simulink model "DDCU_wxt_v03"  (R2014a)
settings: Solver=ode45  StartTime=0.0  StopTime=50  FixedStep=0.0005  RelTol=1e-3
values from neighbouring files (symbols this model uses):
  ag_thr = 0.4*g    (= 3.924)    [Veh_Par_wxt.m]
  B = 2.25    [Veh_Par_wxt.m]
  bra_pre_em = 12    [Veh_Par_wxt.m]
  bra_pre_gz2 = 12/3    (= 4)    [Veh_Par_wxt.m]
  bra_pre_gz34 = 12/3    (= 4)    [Veh_Par_wxt.m]
  bra_pre_yd = 12/2    (= 6)    [Veh_Par_wxt.m]
  brakepre_dem_data = [0 1 2 3 4 5 6 7 8 9 10 11 12]    [Veh_Par_wxt.m]
  brakeTrq_dem_data = [0 218.198 436.396 654.594 872.792 1090.99 1309.188 1527.386 1745.584 1963.782 2181.98 2400.178 2618.376]    [Veh_Par_wxt.m]
  bratrq_max = 4*2618.376    (= 10473.504)    [Veh_Par_wxt.m]
  eff_tran = 0.75    [Veh_Par_wxt.m]
  G = Mass*g    (= 36297)    [Veh_Par_wxt.m]
  kd1 = 1    [Veh_Par_wxt.m]
  kd2 = 1    [Veh_Par_wxt.m]
  kd3 = 1    [Veh_Par_wxt.m]
  ki1 = 1    [Veh_Par_wxt.m]
  ki2 = 1    [Veh_Par_wxt.m]
  ki3 = 1    [Veh_Par_wxt.m]
  kp1 = 1    [Veh_Par_wxt.m]
  kp2 = 1    [Veh_Par_wxt.m]
  kp3 = 1    [Veh_Par_wxt.m]
  L = 3.12    [Veh_Par_wxt.m]
  premax = 12    [Veh_Par_wxt.m]
  Radius = 0.20    (= 0.2)    [Veh_Par_wxt.m]
  s_opt_yi_add = 0.05    [Veh_Par_wxt.m]
  s_opt_zhuan_add = 0.05    [Veh_Par_wxt.m]
  spd_map_mot = [0 100 200 300 360 400 500 600 700 800 900]*tras_ratio    [Veh_Par_wxt.m]
  spdmax = 900*tras_ratio    (= 5580)    [Veh_Par_wxt.m]
  speed_thr_park = 5/3.6/Radius*30/pi    (= 66.3145596216)    [Veh_Par_wxt.m]
  tras_ratio = 6.2    [Veh_Par_wxt.m]
  trq_map_mot = [1200 1200 1200 1200 1200 1080 864 720 617 540 480]/tras_ratio    [Veh_Par_wxt.m]
  trqmax = 80    [Veh_Par_wxt.m]
  v_thr1_b = 5    [Veh_Par_wxt.m]
  v_thr2_b = 20    [Veh_Par_wxt.m]
  v_thr_park = 5    [Veh_Par_wxt.m]
undefined symbols (not defined in the file or in its folder): DiscIntNeverNeededParam
libraries: simulink x34, Solver_SF x1
(part 6 of 10)

== system DDCU_wxt_v03/MainControl/mode_control/backward/backward/Drive/驱动防滑控制TCS/转向TCS/右转 ==
  trq_dem_lf : Inport
  trq_dem_lr : Inport  Port=2
  trq_dem_rf : Inport  Port=3
  trq_dem_rr : Inport  Port=4
  bra_pre_l : Inport  Port=5
  bra_pre_r : Inport  Port=6
  s_act_lf : Inport  Port=7
  s_act_lr : Inport  Port=8
  s_act_rf : Inport  Port=9
  s_act_rr : Inport  Port=10
  brake_dem : Inport  Port=11
  s_opt_zhuan : Inport  Port=12
  Action Port : ActionPort
  Constant{,1..3} (4 alike) : Constant  Value=s_opt_zhuan_add
  MATLAB Function : MATLAB Function  TreatAsAtomicUnit=on
  MATLAB Function1 : MATLAB Function  TreatAsAtomicUnit=on
  MATLAB Function2 : MATLAB Function  TreatAsAtomicUnit=on
  MATLAB Function3 : MATLAB Function  TreatAsAtomicUnit=on
  MATLAB Function4 : MATLAB Function  TreatAsAtomicUnit=on
  Memory{,1..3} (4 alike) : Memory  InheritSampleTime=on
  Multiport Switch : MultiPortSwitch  DataPortOrder=Zero-based contiguous  Inputs=4
  Mux{,1..3} (4 alike) : Mux  Inputs=6
  Switch Case : SwitchCase  CaseConditions={0,1,2,3}  ShowDefaultCase=off
  Terminator : Terminator
  Terminator1 : Terminator
  前后轮均滑转 : Subsystem  TreatAsAtomicUnit=on
  前轮滑转 : Subsystem  TreatAsAtomicUnit=on
  后轮滑转 : Subsystem  TreatAsAtomicUnit=on
  无滑转 : Subsystem  TreatAsAtomicUnit=on
  backward_dem : Outport
  wires:
  s_act_lf/1 -> MATLAB Function/1(s_act_lf), [s_act_lf]
  MATLAB Function/1(flag_lf) -> Memory/1, [flag_lf]
  Memory/1 -> MATLAB Function/4(flag_lf_pre)
  Constant/1 -> MATLAB Function/3(s_opt_zhuan_add)
  s_act_lr/1 -> MATLAB Function1/1(s_act_lr), [s_act_lr]
  MATLAB Function1/1(flag_lr) -> [flag_lr], Memory1/1
  Memory1/1 -> MATLAB Function1/4(flag_lr_pre)
  Constant1/1 -> MATLAB Function1/3(s_opt_zhuan_add)
  s_act_rf/1 -> MATLAB Function2/1(s_act_rf)
  MATLAB Function2/1(flag_rf) -> Memory2/1, Terminator/1
  Memory2/1 -> MATLAB Function2/4(flag_rf_pre)
  Constant2/1 -> MATLAB Function2/3(s_opt_zhuan_add)
  s_act_rr/1 -> MATLAB Function3/1(s_act_rr)
  s_opt_zhuan/1 -> [s_opt_zhuan], MATLAB Function3/2(s_opt_zhuan), MATLAB Function2/2(s_opt_zhuan), MATLAB Function1/2(s_opt_zhuan), MATLAB Function/2(s_opt_zhuan)
  MATLAB Function3/1(flag_rr) -> Memory3/1, Terminator1/1
  Memory3/1 -> MATLAB Function3/4(flag_rr_pre)
  Constant3/1 -> MATLAB Function3/3(s_opt_zhuan_add)
  [flag_lf] -> MATLAB Function4/1(flag_lf)
  [flag_lr] -> MATLAB Function4/2(flag_lr)
  MATLAB Function4/1(y) -> Multiport Switch/1, Switch Case/1
  Switch Case/1 -> 无滑转/Action
  trq_dem_lf/1 -> 无滑转/1(trq_dem_lf), 前后轮均滑转/1(trq_dem_lf), 后轮滑转/1(trq_dem_lf), 前轮滑转/1(trq_dem_lf)
  trq_dem_lr/1 -> 无滑转/2(trq_dem_lr), 前轮滑转/2(trq_dem_lr), 前后轮均滑转/2(trq_dem_lr), 后轮滑转/2(trq_dem_lr)
  trq_dem_rf/1 -> 无滑转/3(trq_dem_rf), 前后轮均滑转/3(trq_dem_rf), 后轮滑转/3(trq_dem_rf), 前轮滑转/3(trq_dem_rf)
  trq_dem_rr/1 -> 无滑转/4(trq_dem_rr), 前后轮均滑转/4(trq_dem_rr), 后轮滑转/4(trq_dem_rr), 前轮滑转/4(trq_dem_rr)
  bra_pre_l/1 -> 无滑转/5(bra_pre_l), 前后轮均滑转/5(bra_pre_l), 后轮滑转/5(bra_pre_l), 前轮滑转/5(bra_pre_l)
  bra_pre_r/1 -> 无滑转/6(bra_pre_r), 前后轮均滑转/6(bra_pre_r), 后轮滑转/6(bra_pre_r), 前轮滑转/6(bra_pre_r)
  brake_dem/1 -> 无滑转/7(brake_dem), 前后轮均滑转/7(brake_dem), 后轮滑转/7(brake_dem), 前轮滑转/7(brake_dem)
  无滑转/1(mot_lf) -> Mux/1
  无滑转/2(mot_lr) -> Mux/2
  无滑转/4(mot_rr) -> Mux/4
  无滑转/3(mot_rf) -> Mux/3
  无滑转/5(bra_pre_l1) -> Mux/5
  无滑转/6(bra_pre_r1) -> Mux/6
  Mux/1 -> Multiport Switch/2
  Multiport Switch/1 -> backward_dem/1
  Switch Case/2 -> 前轮滑转/Action
  前轮滑转/6(bra_pre_r1) -> Mux1/6
  前轮滑转/3(mot_rf) -> Mux1/3
  前轮滑转/2(mot_lr) -> Mux1/2
  前轮滑转/1(mot_lf) -> Mux1/1
  前轮滑转/5(bra_pre_l1) -> Mux1/5
  前轮滑转/4(mot_rr) -> Mux1/4
  Mux1/1 -> Multiport Switch/3
  [s_act_lf] -> 前轮滑转/8(s_act_lf)
  [s_opt_zhuan] -> 前轮滑转/9(s_opt_zhuan)
  后轮滑转/1(mot_lf) -> Mux2/1
  后轮滑转/3(mot_rf) -> Mux2/3
  后轮滑转/2(mot_lr) -> Mux2/2
  后轮滑转/4(mot_rr) -> Mux2/4
  后轮滑转/5(bra_pre_l1) -> Mux2/5
  后轮滑转/6(bra_pre_r1) -> Mux2/6
  Mux2/1 -> Multiport Switch/4
  [s_act_lr] -> 后轮滑转/8(s_act_lr)
  [s_opt_zhuan] -> 后轮滑转/9(s_opt_zhuan)
  Switch Case/3 -> 后轮滑转/Action
  前后轮均滑转/1(mot_lf) -> Mux3/1
  前后轮均滑转/3(mot_rf) -> Mux3/3
  前后轮均滑转/2(mot_lr) -> Mux3/2
  前后轮均滑转/4(mot_rr) -> Mux3/4
  前后轮均滑转/5(bra_pre_l1) -> Mux3/5
  前后轮均滑转/6(bra_pre_r1) -> Mux3/6
  Switch Case/4 -> 前后轮均滑转/Action
  [s_act_lf] -> 前后轮均滑转/8(s_act_lf)
  [s_act_lr] -> 前后轮均滑转/9(s_act_lr)
  [s_opt_zhuan] -> 前后轮均滑转/10(s_opt_zhuan)
  Mux3/1 -> Multiport Switch/5

== system DDCU_wxt_v03/MainControl/mode_control/backward/backward/Drive/驱动防滑控制TCS/转向TCS/左转 ==
  trq_dem_lf : Inport
  trq_dem_lr : Inport  Port=2
  trq_dem_rf : Inport  Port=3
  trq_dem_rr : Inport  Port=4
  bra_pre_l : Inport  Port=5
  bra_pre_r : Inport  Port=6
  s_act_lf : Inport  Port=7
  s_act_lr : Inport  Port=8
  s_act_rf : Inport  Port=9
  s_act_rr : Inport  Port=10
  brake_dem : Inport  Port=11
  s_opt_zhuan : Inport  Port=12
  Action Port : ActionPort
  Constant{,1..3} (4 alike) : Constant  Value=s_opt_zhuan_add
  MATLAB Function : MATLAB Function  TreatAsAtomicUnit=on
  MATLAB Function1 : MATLAB Function  TreatAsAtomicUnit=on
  MATLAB Function2 : MATLAB Function  TreatAsAtomicUnit=on
  MATLAB Function3 : MATLAB Function  TreatAsAtomicUnit=on
  MATLAB Function4 : MATLAB Function  TreatAsAtomicUnit=on
  Memory{,1..3} (4 alike) : Memory  InheritSampleTime=on
  Multiport Switch : MultiPortSwitch  DataPortOrder=Zero-based contiguous  Inputs=4
  Mux{,1..3} (4 alike) : Mux  Inputs=6
  Switch Case : SwitchCase  CaseConditions={0,1,2,3}  ShowDefaultCase=off
  Terminator : Terminator
  Terminator1 : Terminator
  前后轮均滑转 : Subsystem  TreatAsAtomicUnit=on
  前轮滑转 : Subsystem  TreatAsAtomicUnit=on
  后轮滑转 : Subsystem  TreatAsAtomicUnit=on
  无滑转 : Subsystem  TreatAsAtomicUnit=on
  backward_dem : Outport
  wires:
  Mux3/1 -> Multiport Switch/5
  [s_opt_zhuan] -> 前后轮均滑转/10(s_opt_zhuan)
  [s_act_rr] -> 前后轮均滑转/9(s_act_rr)
  [s_act_rf] -> 前后轮均滑转/8(s_act_rf)
  Switch Case/4 -> 前后轮均滑转/Action
  前后轮均滑转/6(bra_pre_r1) -> Mux3/6
  前后轮均滑转/5(bra_pre_l1) -> Mux3/5
  前后轮均滑转/4(mot_rr) -> Mux3/4
  前后轮均滑转/2(mot_lr) -> Mux3/2
  前后轮均滑转/3(mot_rf) -> Mux3/3
  前后轮均滑转/1(mot_lf) -> Mux3/1
  Switch Case/3 -> 后轮滑转/Action
  [s_opt_zhuan] -> 后轮滑转/9(s_opt_zhuan)
  [s_act_rr] -> 后轮滑转/8(s_act_rr)
  Mux2/1 -> Multiport Switch/4
  后轮滑转/6(bra_pre_r1) -> Mux2/6
  后轮滑转/5(bra_pre_l1) -> Mux2/5
  后轮滑转/4(mot_rr) -> Mux2/4
  后轮滑转/2(mot_lr) -> Mux2/2
  后轮滑转/3(mot_rf) -> Mux2/3
  后轮滑转/1(mot_lf) -> Mux2/1
  [s_opt_zhuan] -> 前轮滑转/9(s_opt_zhuan)
  [s_act_rf] -> 前轮滑转/8(s_act_rf)
  Mux1/1 -> Multiport Switch/3
  前轮滑转/4(mot_rr) -> Mux1/4
  前轮滑转/5(bra_pre_l1) -> Mux1/5
  前轮滑转/1(mot_lf) -> Mux1/1
  前轮滑转/2(mot_lr) -> Mux1/2
  前轮滑转/3(mot_rf) -> Mux1/3
  前轮滑转/6(bra_pre_r1) -> Mux1/6
  Switch Case/2 -> 前轮滑转/Action
  Multiport Switch/1 -> backward_dem/1
  Mux/1 -> Multiport Switch/2
  无滑转/6(bra_pre_r1) -> Mux/6
  无滑转/5(bra_pre_l1) -> Mux/5
  无滑转/3(mot_rf) -> Mux/3
  无滑转/4(mot_rr) -> Mux/4
  无滑转/2(mot_lr) -> Mux/2
  无滑转/1(mot_lf) -> Mux/1
  brake_dem/1 -> 前轮滑转/7(brake_dem), 后轮滑转/7(brake_dem), 前后轮均滑转/7(brake_dem), 无滑转/7(brake_dem)
  bra_pre_r/1 -> 前轮滑转/6(bra_pre_r), 后轮滑转/6(bra_pre_r), 前后轮均滑转/6(bra_pre_r), 无滑转/6(bra_pre_r)
  bra_pre_l/1 -> 前轮滑转/5(bra_pre_l), 后轮滑转/5(bra_pre_l), 前后轮均滑转/5(bra_pre_l), 无滑转/5(bra_pre_l)
  trq_dem_rr/1 -> 前轮滑转/4(trq_dem_rr), 后轮滑转/4(trq_dem_rr), 前后轮均滑转/4(trq_dem_rr), 无滑转/4(trq_dem_rr)
  trq_dem_rf/1 -> 前轮滑转/3(trq_dem_rf), 后轮滑转/3(trq_dem_rf), 前后轮均滑转/3(trq_dem_rf), 无滑转/3(trq_dem_rf)
  trq_dem_lr/1 -> 后轮滑转/2(trq_dem_lr), 前后轮均滑转/2(trq_dem_lr), 前轮滑转/2(trq_dem_lr), 无滑转/2(trq_dem_lr)
  trq_dem_lf/1 -> 前轮滑转/1(trq_dem_lf), 后轮滑转/1(trq_dem_lf), 前后轮均滑转/1(trq_dem_lf), 无滑转/1(trq_dem_lf)
  Switch Case/1 -> 无滑转/Action
  MATLAB Function4/1(y) -> Switch Case/1, Multiport Switch/1
  [flag_rr] -> MATLAB Function4/2(flag_rr)
  [flag_rf] -> MATLAB Function4/1(flag_rf)
  Constant3/1 -> MATLAB Function3/3(s_opt_zhuan_add)
  Memory3/1 -> MATLAB Function3/4(flag_rr_pre)
  MATLAB Function3/1(flag_rr) -> Memory3/1, [flag_rr]
  s_opt_zhuan/1 -> MATLAB Function/2(s_opt_zhuan), MATLAB Function1/2(s_opt_zhuan), MATLAB Function2/2(s_opt_zhuan), MATLAB Function3/2(s_opt_zhuan), [s_opt_zhuan]
  s_act_rr/1 -> MATLAB Function3/1(s_act_rr), [s_act_rr]
  Constant2/1 -> MATLAB Function2/3(s_opt_zhuan_add)
  Memory2/1 -> MATLAB Function2/4(flag_rf_pre)
  MATLAB Function2/1(flag_rf) -> [flag_rf], Memory2/1
  s_act_rf/1 -> MATLAB Function2/1(s_act_rf), [s_act_rf]
  Constant1/1 -> MATLAB Function1/3(s_opt_zhuan_add)
  Memory1/1 -> MATLAB Function1/4(flag_lr_pre)
  MATLAB Function1/1(flag_lr) -> Memory1/1, Terminator1/1
  s_act_lr/1 -> MATLAB Function1/1(s_act_lr)
  Constant/1 -> MATLAB Function/3(s_opt_zhuan_add)
  Memory/1 -> MATLAB Function/4(flag_lf_pre)
  MATLAB Function/1(flag_lf) -> Memory/1, Terminator/1
  s_act_lf/1 -> MATLAB Function/1(s_act_lf)

== system DDCU_wxt_v03/MainControl/mode_control/forward/forward/Drive/驱动防滑控制TCS/直行TCS/Subsystem ==
  speed_act_lf : Inport
  v_act : Inport  Port=2
  Add : Sum
  Constant : Constant  Value=eps
  Divide : Product  Inputs=*/
  Gain : Gain  Gain=pi/30
  Gain1 : Gain  Gain=Radius
  Gain2 : Gain  Gain=1/3.6
  Subtract : Sum  Inputs=+-
  s_act_lf : Outport
  wires:
  Divide/1 -> s_act_lf/1
  Add/1 -> Divide/2
  Constant/1 -> Add/2
  Subtract/1 -> Divide/1
  Gain2/1 -> Subtract/2
  Gain1/1 -> Subtract/1, Add/1
  v_act/1 -> Gain2/1
  Gain/1 -> Gain1/1
  speed_act_lf/1 -> Gain/1

== system DDCU_wxt_v03/MainControl/mode_control/forward/forward/Drive/驱动防滑控制TCS/直行TCS/Subsystem1 ==
  speed_act_lr : Inport
  v_act : Inport  Port=2
  Add : Sum
  Constant : Constant  Value=eps
  Divide : Product  Inputs=*/
  Gain : Gain  Gain=pi/30
  Gain1 : Gain  Gain=Radius
  Gain2 : Gain  Gain=1/3.6
  Subtract : Sum  Inputs=+-
  s_act_lr : Outport
  wires:
  speed_act_lr/1 -> Gain/1
  Gain/1 -> Gain1/1
  v_act/1 -> Gain2/1
  Gain1/1 -> Add/1, Subtract/1
  Gain2/1 -> Subtract/2
  Subtract/1 -> Divide/1
  Constant/1 -> Add/2
  Add/1 -> Divide/2
  Divide/1 -> s_act_lr/1

== system DDCU_wxt_v03/MainControl/mode_control/forward/forward/Drive/驱动防滑控制TCS/直行TCS/Subsystem2 ==
  speed_act_rf : Inport
  v_act : Inport  Port=2
  Add : Sum
  Constant : Constant  Value=eps
  Divide : Product  Inputs=*/
  Gain : Gain  Gain=pi/30
  Gain1 : Gain  Gain=Radius
  Gain2 : Gain  Gain=1/3.6
  Subtract : Sum  Inputs=+-
  s_act_rf : Outport
  wires:
  Divide/1 -> s_act_rf/1
  Add/1 -> Divide/2
  Constant/1 -> Add/2
  Subtract/1 -> Divide/1
  Gain2/1 -> Subtract/2
  Gain1/1 -> Subtract/1, Add/1
  v_act/1 -> Gain2/1
  Gain/1 -> Gain1/1
  speed_act_rf/1 -> Gain/1

== system DDCU_wxt_v03/MainControl/mode_control/forward/forward/Drive/驱动防滑控制TCS/直行TCS/Subsystem3 ==
  speed_act_rr : Inport
  v_act : Inport  Port=2
  Add : Sum
  Constant : Constant  Value=eps
  Divide : Product  Inputs=*/
  Gain : Gain  Gain=pi/30
  Gain1 : Gain  Gain=Radius
  Gain2 : Gain  Gain=1/3.6
  Subtract : Sum  Inputs=+-
  s_act_rr : Outport
  wires:
  speed_act_rr/1 -> Gain/1
  Gain/1 -> Gain1/1
  v_act/1 -> Gain2/1
  Gain1/1 -> Add/1, Subtract/1
  Gain2/1 -> Subtract/2
  Subtract/1 -> Divide/1
  Constant/1 -> Add/2
  Add/1 -> Divide/2
  Divide/1 -> s_act_rr/1

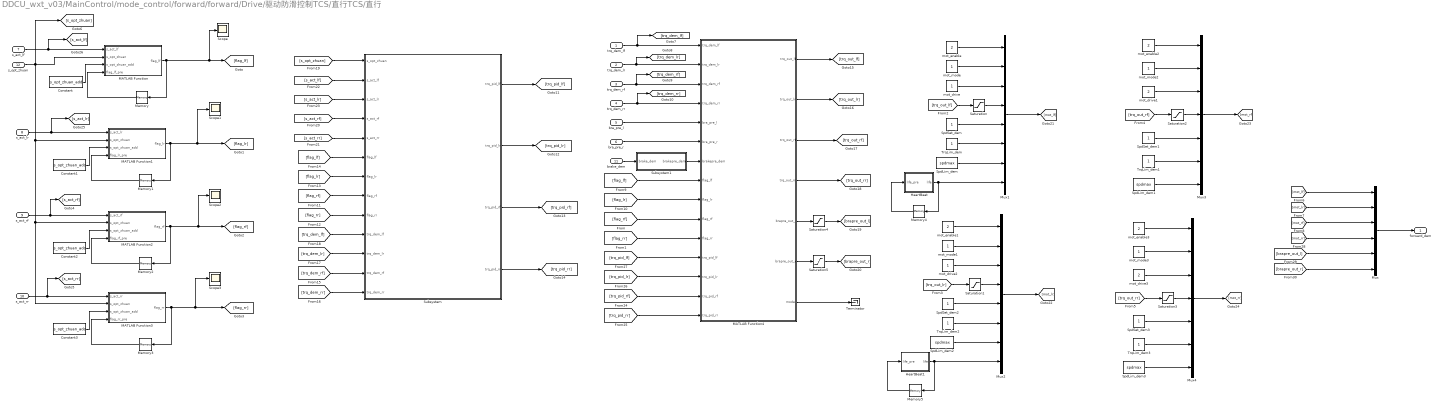
== system DDCU_wxt_v03/MainControl/mode_control/forward/forward/Drive/驱动防滑控制TCS/直行TCS/直行 ==
  trq_dem_lf : Inport
  trq_dem_lr : Inport  Port=2
  trq_dem_rf : Inport  Port=3
  trq_dem_rr : Inport  Port=4
  bra_pre_l : Inport  Port=5
  bra_pre_r : Inport  Port=6
  s_act_lf : Inport  Port=7
  s_act_lr : Inport  Port=8
  s_act_rf : Inport  Port=9
  s_act_rr : Inport  Port=10
  brake_dem : Inport  Port=11
  s_opt_zhuan : Inport  Port=12
  Constant{,1..3} (4 alike) : Constant  Value=s_opt_zhuan_add
  HeartBeat : MATLAB Function  TreatAsAtomicUnit=on
  HeartBeat1 : MATLAB Function  TreatAsAtomicUnit=on
  MATLAB Function : MATLAB Function  TreatAsAtomicUnit=on
  MATLAB Function1 : MATLAB Function  TreatAsAtomicUnit=on
  MATLAB Function2 : MATLAB Function  TreatAsAtomicUnit=on
  MATLAB Function3 : MATLAB Function  TreatAsAtomicUnit=on
  MATLAB Function4 : MATLAB Function  TreatAsAtomicUnit=on
  Memory{,1..5} (6 alike) : Memory  InheritSampleTime=on
  Mux : Mux  Inputs=6
  Mux1 : Mux  Inputs=8
  Mux2 : Mux  Inputs=8
  Mux3 : Mux  Inputs=7
  Mux4 : Mux  Inputs=7
  Saturation{,1..3} (4 alike) : Saturate  UpperLimit=trqmax  LowerLimit=0
  Saturation4 : Saturate  UpperLimit=premax  LowerLimit=0
  Saturation5 : Saturate  UpperLimit=premax  LowerLimit=0
  Scope{,1..3} (4 alike) : Scope
      Scope settings: SaveName=ScopeData43
      Scope1 settings: SaveName=ScopeData44
      Scope2 settings: SaveName=ScopeData45
      Scope3 settings: SaveName=ScopeData46
  SpdLim_dem{,1..3} (4 alike) : Constant  Value=spdmax
  SpdSet_dem{,1..3} (4 alike) : Constant
  Subsystem : Subsystem
  Subsystem1 : Subsystem
  Terminator : Terminator
  TrqLim_dem{,1..3} (4 alike) : Constant
  mot_drive : Constant
  mot_drive1 : Constant  Value=2
  mot_drive2 : Constant
  mot_drive3 : Constant  Value=2
  mot_enable{,1..3} (4 alike) : Constant  Value=2
  mot_mode{,1..3} (4 alike) : Constant
  forward_dem : Outport
  wires:
  Mux/1 -> forward_dem/1
  [flag_rr] -> MATLAB Function4/11(flag_rr)
  [flag_rf] -> MATLAB Function4/10(flag_rf)
  Constant3/1 -> MATLAB Function3/3(s_opt_zhuan_add)
  Memory3/1 -> MATLAB Function3/4(flag_rr_pre)
  MATLAB Function3/1(flag_rr) -> Memory3/1, Scope3/1, [flag_rr]
  s_opt_zhuan/1 -> MATLAB Function/2(s_opt_zhuan), MATLAB Function1/2(s_opt_zhuan), MATLAB Function2/2(s_opt_zhuan), MATLAB Function3/2(s_opt_zhuan), [s_opt_zhuan]
  s_act_rr/1 -> MATLAB Function3/1(s_act_rr), [s_act_rr]
  Constant2/1 -> MATLAB Function2/3(s_opt_zhuan_add)
  Memory2/1 -> MATLAB Function2/4(flag_rf_pre)
  MATLAB Function2/1(flag_rf) -> Scope2/1, [flag_rf], Memory2/1
  s_act_rf/1 -> MATLAB Function2/1(s_act_rf), [s_act_rf]
  Constant1/1 -> MATLAB Function1/3(s_opt_zhuan_add)
  Memory1/1 -> MATLAB Function1/4(flag_lr_pre)
  MATLAB Function1/1(flag_lr) -> Memory1/1, Scope1/1, [flag_lr]
  s_act_lr/1 -> [s_act_lr], MATLAB Function1/1(s_act_lr)
  Constant/1 -> MATLAB Function/3(s_opt_zhuan_add)
  Memory/1 -> MATLAB Function/4(flag_lf_pre)
  MATLAB Function/1(flag_lf) -> Scope/1, [flag_lf], Memory/1
  s_act_lf/1 -> [s_act_lf], MATLAB Function/1(s_act_lf)
  [flag_lr] -> MATLAB Function4/9(flag_lr)
  [flag_lf] -> MATLAB Function4/8(flag_lf)
  [trq_dem_lf] -> Subsystem/10(trq_dem_lf)
  [flag_lf] -> Subsystem/6(flag_lf)
  [trq_dem_rf] -> Subsystem/12(trq_dem_rf)
  [trq_dem_lr] -> Subsystem/11(trq_dem_lr)
  [flag_lr] -> Subsystem/7(flag_lr)
  [flag_rf] -> Subsystem/8(flag_rf)
  [trq_dem_rr] -> Subsystem/13(trq_dem_rr)
  [flag_rr] -> Subsystem/9(flag_rr)
  [s_opt_zhuan] -> Subsystem/1(s_opt_zhuan)
  [s_act_rr] -> Subsystem/5(s_act_rr)
  [s_act_rf] -> Subsystem/4(s_act_rf)
  [s_act_lr] -> Subsystem/3(s_act_lr)
  [s_act_lf] -> Subsystem/2(s_act_lf)
  Subsystem/2(trq_pid_lr) -> [trq_pid_lr]
  Subsystem/1(trq_pid_lf) -> [trq_pid_lf]
  Subsystem/4(trq_pid_rr) -> [trq_pid_rr]
  Subsystem/3(trq_pid_rf) -> [trq_pid_rf]
  [trq_pid_lf] -> MATLAB Function4/12(trq_pid_lf)
  [trq_pid_lr] -> MATLAB Function4/13(trq_pid_lr)
  [trq_pid_rf] -> MATLAB Function4/14(trq_pid_rf)
  [trq_pid_rr] -> MATLAB Function4/15(trq_pid_rr)
  trq_dem_lf/1 -> MATLAB Function4/1(trq_dem_lf), [trq_dem_lf]
  trq_dem_lr/1 -> MATLAB Function4/2(trq_dem_lr), [trq_dem_lr]
  trq_dem_rf/1 -> MATLAB Function4/3(trq_dem_rf), [trq_dem_rf]
  trq_dem_rr/1 -> MATLAB Function4/4(trq_dem_rr), [trq_dem_rr]
  bra_pre_l/1 -> MATLAB Function4/5(bra_pre_l)
  bra_pre_r/1 -> MATLAB Function4/6(bra_pre_r)
  SpdLim_dem3/1 -> Mux4/7
  TrqLim_dem3/1 -> Mux4/6
  Mux4/1 -> [mot_rr]
  SpdSet_dem3/1 -> Mux4/5
  mot_enable3/1 -> Mux4/1
  [trq_out_rr] -> Saturation3/1
  mot_mode3/1 -> Mux4/2
  mot_drive3/1 -> Mux4/3
  SpdLim_dem2/1 -> Mux2/7
  Memory5/1 -> HeartBeat1/1(life_pre)
  HeartBeat1/1(life) -> Memory5/1, Mux2/8
  TrqLim_dem2/1 -> Mux2/6
  Mux2/1 -> [mot_lr]
  SpdSet_dem2/1 -> Mux2/5
  mot_enable1/1 -> Mux2/1
  [trq_out_lr] -> Saturation1/1
  mot_mode1/1 -> Mux2/2
  mot_drive2/1 -> Mux2/3
  SpdLim_dem1/1 -> Mux3/7
  TrqLim_dem1/1 -> Mux3/6
  Mux3/1 -> [mot_rf]
  SpdSet_dem1/1 -> Mux3/5
  mot_enable2/1 -> Mux3/1
  [trq_out_rf] -> Saturation2/1
  mot_mode2/1 -> Mux3/2
  mot_drive1/1 -> Mux3/3
  SpdLim_dem/1 -> Mux1/7
  Memory4/1 -> HeartBeat/1(life_pre)
  HeartBeat/1(life) -> Memory4/1, Mux1/8
  TrqLim_dem/1 -> Mux1/6
  Mux1/1 -> [mot_lf]
  SpdSet_dem/1 -> Mux1/5
  mot_enable/1 -> Mux1/1
  [trq_out_lf] -> Saturation/1
  mot_mode/1 -> Mux1/2
  mot_drive/1 -> Mux1/3
  MATLAB Function4/1(trq_out_lf) -> [trq_out_lf]
  MATLAB Function4/2(trq_out_lr) -> [trq_out_lr]
  MATLAB Function4/3(trq_out_rf) -> [trq_out_rf]
  MATLAB Function4/4(trq_out_rr) -> [trq_out_rr]
  MATLAB Function4/5(brapre_out_l) -> Saturation4/1
  MATLAB Function4/6(brapre_out_r) -> Saturation5/1
  [mot_lf] -> Mux/1
  [mot_lr] -> Mux/2
  [mot_rf] -> Mux/3
  [mot_rr] -> Mux/4
  [brapre_out_l] -> Mux/5
  [brapre_out_r] -> Mux/6
  Subsystem1/1(brakepre_dem) -> MATLAB Function4/7(brakepre_dem)
  brake_dem/1 -> Subsystem1/1(brake_dem)
  MATLAB Function4/7(mode) -> Terminator/1
  Saturation/1 -> Mux1/4
  Saturation2/1 -> Mux3/4
  Saturation1/1 -> Mux2/4
  Saturation3/1 -> Mux4/4
  Saturation4/1 -> [brapre_out_l]
  Saturation5/1 -> [brapre_out_r]

== system DDCU_wxt_v03/MainControl/mode_control/forward/forward/Drive/驱动防滑控制TCS/转向TCS/Subsystem ==
  speed_act_lf : Inport
  v_act : Inport  Port=2
  Add : Sum
  Constant : Constant  Value=eps
  Divide : Product  Inputs=*/
  Gain : Gain  Gain=pi/30
  Gain1 : Gain  Gain=Radius
  Gain2 : Gain  Gain=1/3.6
  Subtract : Sum  Inputs=+-
  s_act_lf : Outport
  wires:
  speed_act_lf/1 -> Gain/1
  Gain/1 -> Gain1/1
  v_act/1 -> Gain2/1
  Gain1/1 -> Add/1, Subtract/1
  Gain2/1 -> Subtract/2
  Subtract/1 -> Divide/1
  Constant/1 -> Add/2
  Add/1 -> Divide/2
  Divide/1 -> s_act_lf/1

== system DDCU_wxt_v03/MainControl/mode_control/forward/forward/Drive/驱动防滑控制TCS/转向TCS/Subsystem1 ==
  speed_act_lr : Inport
  v_act : Inport  Port=2
  Add : Sum
  Constant : Constant  Value=eps
  Divide : Product  Inputs=*/
  Gain : Gain  Gain=pi/30
  Gain1 : Gain  Gain=Radius
  Gain2 : Gain  Gain=1/3.6
  Subtract : Sum  Inputs=+-
  s_act_lr : Outport
  wires:
  Divide/1 -> s_act_lr/1
  Add/1 -> Divide/2
  Constant/1 -> Add/2
  Subtract/1 -> Divide/1
  Gain2/1 -> Subtract/2
  Gain1/1 -> Subtract/1, Add/1
  v_act/1 -> Gain2/1
  Gain/1 -> Gain1/1
  speed_act_lr/1 -> Gain/1

== system DDCU_wxt_v03/MainControl/mode_control/forward/forward/Drive/驱动防滑控制TCS/转向TCS/Subsystem2 ==
  speed_act_rf : Inport
  v_act : Inport  Port=2
  Add : Sum
  Constant : Constant  Value=eps
  Divide : Product  Inputs=*/
  Gain : Gain  Gain=pi/30
  Gain1 : Gain  Gain=Radius
  Gain2 : Gain  Gain=1/3.6
  Subtract : Sum  Inputs=+-
  s_act_rf : Outport
  wires:
  speed_act_rf/1 -> Gain/1
  Gain/1 -> Gain1/1
  v_act/1 -> Gain2/1
  Gain1/1 -> Add/1, Subtract/1
  Gain2/1 -> Subtract/2
  Subtract/1 -> Divide/1
  Constant/1 -> Add/2
  Add/1 -> Divide/2
  Divide/1 -> s_act_rf/1

== system DDCU_wxt_v03/MainControl/mode_control/forward/forward/Drive/驱动防滑控制TCS/转向TCS/Subsystem3 ==
  speed_act_rr : Inport
  v_act : Inport  Port=2
  Add : Sum
  Constant : Constant  Value=eps
  Divide : Product  Inputs=*/
  Gain : Gain  Gain=pi/30
  Gain1 : Gain  Gain=Radius
  Gain2 : Gain  Gain=1/3.6
  Subtract : Sum  Inputs=+-
  s_act_rr : Outport
  wires:
  Divide/1 -> s_act_rr/1
  Add/1 -> Divide/2
  Constant/1 -> Add/2
  Subtract/1 -> Divide/1
  Gain2/1 -> Subtract/2
  Gain1/1 -> Subtract/1, Add/1
  v_act/1 -> Gain2/1
  Gain/1 -> Gain1/1
  speed_act_rr/1 -> Gain/1

== matlab function DDCU_wxt_v03/MainControl/mode_control/backward/backward/Drive/目标转向力矩确定模块/MATLAB Function1 ==
  data: v_act input; Rturn_min_ag output; ag_thr input
function Rturn_min_ag = fcn(v_act,ag_thr)
%#codegen

    Rturn_min_ag=(v_act/3.6)^2/ag_thr;
end

== matlab function DDCU_wxt_v03/MainControl/mode_control/backward/backward/Drive/目标转向力矩确定模块/MATLAB Function2 ==
  data: umax input; delta_Tsteer_max output; G input; L input; B input; Radius input; Rturn_min_xy input
function delta_Tsteer_max = fcn(umax,G,L,B,Radius,Rturn_min_xy)
%#codegen

    delta_Fsteer_max=umax/(0.925+0.15*(Rturn_min_xy/B))*G*L/(2*B);
    delta_Tsteer_max=delta_Fsteer_max*Radius;
    
end

== matlab function DDCU_wxt_v03/MainControl/mode_control/backward/backward/Drive/驱动防滑控制TCS/直行TCS/直行/HeartBeat1 ==
  data: life_pre input; life output
function life = fcn(life_pre)
%#codegen
life=life_pre+1;
if life>15
    life=0;
end
end

== matlab function DDCU_wxt_v03/MainControl/mode_control/backward/backward/Drive/驱动防滑控制TCS/直行TCS/直行/MATLAB Function3 ==
  data: s_act_rr input; flag_rr output; s_opt_zhuan input; s_opt_zhuan_add input; flag_rr_pre input
function flag_rr = fcn(s_act_rr,s_opt_zhuan,s_opt_zhuan_add,flag_rr_pre)
%#codegen
if s_act_rr>s_opt_zhuan+s_opt_zhuan_add
    flag_rr=1;
elseif s_act_rr<s_opt_zhuan
    flag_rr = 0;
else
    flag_rr=flag_rr_pre;
end
end

== matlab function DDCU_wxt_v03/MainControl/mode_control/backward/backward/Drive/驱动防滑控制TCS/转向TCS/右转/MATLAB Function2 ==
  data: s_act_rf input; flag_rf output; s_opt_zhuan input; s_opt_zhuan_add input; flag_rf_pre input
function flag_rf = fcn(s_act_rf,s_opt_zhuan,s_opt_zhuan_add,flag_rf_pre)
%#codegen
if s_act_rf>s_opt_zhuan+s_opt_zhuan_add
    flag_rf=1;
elseif s_act_rf<s_opt_zhuan
    flag_rf = 0;
else
    flag_rf=flag_rf_pre;
end
end

== matlab function DDCU_wxt_v03/MainControl/mode_control/backward/backward/Drive/驱动防滑控制TCS/转向TCS/右转/前后轮均滑转/HeartBeat1 ==
  data: life_pre input; life output
function life = fcn(life_pre)
%#codegen
life=life_pre+1;
if life>15
    life=0;
end
end

== matlab function DDCU_wxt_v03/MainControl/mode_control/backward/backward/Drive/驱动防滑控制TCS/转向TCS/右转/后轮滑转/HeartBeat ==
  data: life_pre input; life output
function life = fcn(life_pre)
%#codegen
life=life_pre+1;
if life>15
    life=0;
end
end

== matlab function DDCU_wxt_v03/MainControl/mode_control/backward/backward/Drive/驱动防滑控制TCS/转向TCS/左转/MATLAB Function ==
  data: s_act_lf input; flag_lf output; s_opt_zhuan input; s_opt_zhuan_add input; flag_lf_pre input
function flag_lf = fcn(s_act_lf,s_opt_zhuan,s_opt_zhuan_add,flag_lf_pre)
%#codegen
if s_act_lf>s_opt_zhuan+s_opt_zhuan_add
    flag_lf=1;
elseif s_act_lf<s_opt_zhuan
    flag_lf = 0;
else
    flag_lf=flag_lf_pre;
end
end

== matlab function DDCU_wxt_v03/MainControl/mode_control/backward/backward/Drive/驱动防滑控制TCS/转向TCS/左转/MATLAB Function4 ==
  data: y output; flag_rf input; flag_rr input
function y = fcn(flag_rf,flag_rr)
%#codegen只判断外侧车轮滑转状况，不能满足要求再进一步修改。
if flag_rf==0 && flag_rr==0
    y=0;
elseif flag_rf==1 && flag_rr==0
    y=1;
elseif flag_rf==0 && flag_rr==1
    y=2;
else
    %     flag_rf==1 && flag_rr==1
    y=3;
end
end

== matlab function DDCU_wxt_v03/MainControl/mode_control/backward/backward/Drive/驱动防滑控制TCS/转向TCS/左转/后轮滑转/HeartBeat1 ==
  data: life_pre input; life output
function life = fcn(life_pre)
%#codegen
life=life_pre+1;
if life>15
    life=0;
end
end

== matlab function DDCU_wxt_v03/MainControl/mode_control/backward/backward/MATLAB Function ==
  data: acc_dem input; y output; brake_dem input; HAC input
function y = fcn(acc_dem,brake_dem,HAC)
%#codegen
if HAC==1
    if acc_dem>0
        y=0;
    else
        y=1;
    end
else
    if brake_dem==0
        y=0;
    else
        y=1;
    end
end
end

== matlab function DDCU_wxt_v03/MainControl/mode_control/emergency_stop/emergency_stop/HeartBeat ==
  data: life_pre input; life output
function life = fcn(life_pre)
%#codegen
life=life_pre+1;
if life>15
    life=0;
end
end

== matlab function DDCU_wxt_v03/MainControl/mode_control/forward/forward/Brake/HeartBeat ==
  data: life_pre input; life output
function life = fcn(life_pre)
%#codegen
life=life_pre+1;
if life>15
    life=0;
end
end

== matlab function DDCU_wxt_v03/MainControl/mode_control/forward/forward/Brake/MATLAB Function ==
  data: guzhang_lf input; gz_total output; guzhang_lr input; guzhang_rf input; guzhang_rr input
function gz_total = fcn(guzhang_lf,guzhang_lr,guzhang_rf,guzhang_rr)
%#codegen
if guzhang_lf==0 && guzhang_lr==0 && guzhang_rf==0 && guzhang_rr==0
    gz_total=0;
else
    gz_total=1;
end
end

== matlab function DDCU_wxt_v03/MainControl/mode_control/forward/forward/Brake/MATLAB Function2 ==
  data: syi_act_lr input; flagyi_lr output; s_opt_yi input; s_opt_yi_add input; flagyi_lr_pre input
function flagyi_lr = fcn(syi_act_lr,s_opt_yi,s_opt_yi_add,flagyi_lr_pre)
%#codegen
if syi_act_lr>s_opt_yi+s_opt_yi_add
    flagyi_lr=1;
elseif syi_act_lr<s_opt_yi
    flagyi_lr = 0;
else
    flagyi_lr=flagyi_lr_pre;
end
end

== matlab function DDCU_wxt_v03/MainControl/mode_control/forward/forward/Brake/MATLAB Function4 ==
  data: syi_act_rr input; flagyi_rr output; s_opt_yi input; s_opt_yi_add input; flagyi_rr_pre input
function flagyi_rr = fcn(syi_act_rr,s_opt_yi,s_opt_yi_add,flagyi_rr_pre)
%#codegen
if syi_act_rr>s_opt_yi+s_opt_yi_add
    flagyi_rr=1;
elseif syi_act_rr<s_opt_yi
    flagyi_rr = 0;
else
    flagyi_rr=flagyi_rr_pre;
end
end

== matlab function DDCU_wxt_v03/MainControl/mode_control/forward/forward/Drive/MATLAB Function ==
  data: acc_y input; y output; steer_dem input; ag_thr input
function y = fcn(acc_y,steer_dem,ag_thr)
%#codegen
if abs(acc_y)>=ag_thr
    y=0;
elseif steer_dem~=0
    y=1;
else 
    y=2;
end
end

== matlab function DDCU_wxt_v03/MainControl/mode_control/forward/forward/Drive/容错控制/MATLAB Function ==
  data: trq_dem_l input; trq_dem_lf output; trq_dem_r input; trqlim_lf input; trqlim_lr input; trqlim_rf input; trqlim_rr input; guzhang_lf input; guzhang_lr input; guzhang_rf input; guzhang_rr input; trq_dem_lr output; trq_dem_rf output; trq_dem_rr output; bra_pre_l output; bra_pre_r output; bra_pre_gz2 input; bra_pre_gz34 input; mode output
 function [trq_dem_lf,trq_dem_lr,trq_dem_rf,trq_dem_rr,bra_pre_l,bra_pre_r,mode] = fcn(trq_dem_l,trq_dem_r,trqlim_lf,trqlim_lr,trqlim_rf,trqlim_rr,guzhang_lf,guzhang_lr,guzhang_rf,guzhang_rr,bra_pre_gz2,bra_pre_gz34)
%#codegen
if guzhang_lf==0 && guzhang_lr==0 && guzhang_rf==0 && guzhang_rr==0    %0电机故障,平均分配
    trq_dem_lf=trq_dem_l/2;
    trq_dem_lr=trq_dem_l/2;
    trq_dem_rf=trq_dem_r/2;
    trq_dem_rr=trq_dem_r/2;
    bra_pre_l=0;
    bra_pre_r=0;
    mode=1;
elseif  guzhang_lf==1 && guzhang_lr==0 && guzhang_rf==0 && guzhang_rr==0  %1电机故障，同侧电机进行力矩转移，超过限值后，对侧亦降扭。
    trq_dem_lf=0;
    trq_dem_lr=min(trq_dem_l,trqlim_lr);
    trq_dem_rf=(trq_dem_r-(trq_dem_l-trq_dem_lr))/2;
    trq_dem_rr=(trq_dem_r-(trq_dem_l-trq_dem_lr))/2;
    bra_pre_l=0;
    bra_pre_r=0;
    mode=2;
elseif  guzhang_lf==0 && guzhang_lr==1 && guzhang_rf==0 && guzhang_rr==0
    trq_dem_lf=min(trq_dem_l,trqlim_lf);
    trq_dem_lr=0;
    trq_dem_rf=(trq_dem_r-(trq_dem_l-trq_dem_lf))/2;
    trq_dem_rr=(trq_dem_r-(trq_dem_l-trq_dem_lf))/2;
    bra_pre_l=0;
    bra_pre_r=0;
    mode=3;
elseif  guzhang_lf==0 && guzhang_lr==0 && guzhang_rf==1 && guzhang_rr==0
    trq_dem_rf=0;
    trq_dem_rr=min(trq_dem_r,trqlim_rr);
    trq_dem_lf=(trq_dem_l-(trq_dem_r-trq_dem_rr))/2;
    trq_dem_lr=(trq_dem_l-(trq_dem_r-trq_dem_rr))/2;
    bra_pre_l=0;
    bra_pre_r=0;
    mode=4;
elseif  guzhang_lf==0 && guzhang_lr==0 && guzhang_rf==0 && guzhang_rr==1
    trq_dem_rf=min(trq_dem_r,trqlim_rf);
    trq_dem_rr=0;
    trq_dem_lf=(trq_dem_l-(trq_dem_r-trq_dem_rf))/2;
    trq_dem_lr=(trq_dem_l-(trq_dem_r-trq_dem_rf))/2;
    bra_pre_l=0;
    bra_pre_r=0;
    mode=5;
elseif  (guzhang_lf==1 && guzhang_lr==1 && guzhang_rf==0 && guzhang_rr==0) || (guzhang_lf==0 && guzhang_lr==0 && guzhang_rf==1 && guzhang_rr==1) %2电机故障，同侧电机故障,电机目标力矩全部置0，并施加制动直至停车
    trq_dem_rf=0;
    trq_dem_rr=0;
    trq_dem_lf=0;
    trq_dem_lr=0;
    bra_pre_l=bra_pre_gz2;
    bra_pre_r=bra_pre_gz2;
    mode=6;
elseif  guzhang_lf==1 && guzhang_lr==0 && guzhang_rf==1 && guzhang_rr==0 %2电机故障，对侧双电机故障,有4种情况,前两电机故障
    trq_dem_lf=0;
    trq_dem_rf=0;
    if trq_dem_l>=trq_dem_r
        trq_dem_lr=min(trq_dem_l,trqlim_lr);
        trq_dem_rr=min(min(trq_dem_r,trqlim_rr),(trq_dem_r-(trq_dem_l-trq_dem_lr)));
    else
        trq_dem_rr=min(trq_dem_r,trqlim_rr);
        trq_dem_lr=min(min(trq_dem_l,trqlim_lr),(trq_dem_l-(trq_dem_r-trq_dem_rr)));
    end
    bra_pre_l=0;
    bra_pre_r=0;
    mode=8;
elseif  guzhang_lf==0 && guzhang_lr==1 && guzhang_rf==0 && guzhang_rr==1 %后两电机故障
    trq_dem_lr=0;
    trq_dem_rr=0;
    if trq_dem_l>=trq_dem_r
        trq_dem_lf=min(trq_dem_l,trqlim_lf);
        trq_dem_rf=min(min(trq_dem_r,trqlim_rf),(trq_dem_r-(trq_dem_l-trq_dem_lf)));
    else
        trq_dem_rf=min(trq_dem_r,trqlim_rf);
        trq_dem_lf=min(min(trq_dem_l,trqlim_lf),(trq_dem_l-(trq_dem_r-trq_dem_rf)));
    end
    bra_pre_l=0;
    bra_pre_r=0;
    mode=9;
elseif  guzhang_lf==1 && guzhang_lr==0 && guzhang_rf==0 && guzhang_rr==1 %左前电机和右后电机故障
    trq_dem_lf=0;
    trq_dem_rr=0;
    if trq_dem_l>=trq_dem_r
        trq_dem_lr=min(trq_dem_l,trqlim_lr);
        trq_dem_rf=min(min(trq_dem_r,trqlim_rf),(trq_dem_r-(trq_dem_l-trq_dem_lr)));
    else
        trq_dem_rf=min(trq_dem_r,trqlim_rf);
        trq_dem_lr=min(min(trq_dem_l,trqlim_lr),(trq_dem_l-(trq_dem_r-trq_dem_rf)));
    end
    bra_pre_l=0;
    bra_pre_r=0;
    mode=10;
elseif  guzhang_lf==0 && guzhang_lr==1 && guzhang_rf==1 && guzhang_rr==0 %左后电机和右前电机故障
    trq_dem_lr=0;
    trq_dem_rf=0;
    if trq_dem_l>=trq_dem_r
        trq_dem_lf=min(trq_dem_l,trqlim_lf);
        trq_dem_rr=min(min(trq_dem_r,trqlim_rr),(trq_dem_r-(trq_dem_l-trq_dem_lf)));
    else
        trq_dem_rr=min(trq_dem_r,trqlim_rr);
        trq_dem_lf=min(min(trq_dem_l,trqlim_lf),(trq_dem_l-(trq_dem_r-trq_dem_rr)));
    end
    bra_pre_l=0;
    bra_pre_r=0;
    mode=11;
else
    %     (guzhang_lf==1 && guzhang_lr==1 && guzhang_rf==1 && guzhang_rr==0) || (guzhang_lf==1 && guzhang_lr==1 && guzhang_rf==0 && guzhang_rr==1) || (guzhang_lf==1 && guzhang_lr==0 && guzhang_rf==1 && guzhang_rr==1) || (guzhang_lf==0 && guzhang_lr==1 && guzhang_rf==1 && guzhang_rr==1) || (guzhang_lf==1 && guzhang_lr==1 && guzhang_rf==1 && guzhang_rr==1)
    % 三电机或者四电机故障
    trq_dem_rf=0;
    trq_dem_rr=0;
    trq_dem_lf=0;
    trq_dem_lr=0;
    bra_pre_l=bra_pre_gz34;
    bra_pre_r=bra_pre_gz34;
    mode=12;
end
% trq_dem_lf=max(0,trq_dem_lf);%电机转矩不小于0，就是不能出现负值
% trq_dem_lr=max(0,trq_dem_lr);
% trq_dem_rf=max(0,trq_dem_rf);
% trq_dem_rr=max(0,trq_dem_rr);
trq_dem_lf=max(-trqlim_lf,trq_dem_lf);%电机转矩可以出现负值，不超过负的外特性
trq_dem_lr=max(-trqlim_lr,trq_dem_lr);
trq_dem_rf=max(-trqlim_rf,trq_dem_rf);
trq_dem_rr=max(-trqlim_rr,trq_dem_rr);
bra_pre_l=bra_pre_l;
bra_pre_r=bra_pre_r;
end

== matlab function DDCU_wxt_v03/MainControl/mode_control/forward/forward/Drive/驱动防滑控制TCS/转向TCS/右转/MATLAB Function1 ==
  data: s_act_lr input; flag_lr output; s_opt_zhuan input; s_opt_zhuan_add input; flag_lr_pre input
function flag_lr = fcn(s_act_lr,s_opt_zhuan,s_opt_zhuan_add,flag_lr_pre)
%#codegen
if s_act_lr>s_opt_zhuan+s_opt_zhuan_add
    flag_lr=1;
elseif s_act_lr<s_opt_zhuan
    flag_lr = 0;
else
    flag_lr=flag_lr_pre;
end
end

== matlab function DDCU_wxt_v03/MainControl/mode_control/forward/forward/Drive/驱动防滑控制TCS/转向TCS/右转/MATLAB Function3 ==
  data: s_act_rr input; flag_rr output; s_opt_zhuan input; s_opt_zhuan_add input; flag_rr_pre input
function flag_rr = fcn(s_act_rr,s_opt_zhuan,s_opt_zhuan_add,flag_rr_pre)
%#codegen
if s_act_rr>s_opt_zhuan+s_opt_zhuan_add
    flag_rr=1;
elseif s_act_rr<s_opt_zhuan
    flag_rr = 0;
else
    flag_rr=flag_rr_pre;
end
end

== matlab function DDCU_wxt_v03/MainControl/mode_control/forward/forward/Drive/驱动防滑控制TCS/转向TCS/右转/前后轮均滑转/HeartBeat ==
  data: life_pre input; life output
function life = fcn(life_pre)
%#codegen
life=life_pre+1;
if life>15
    life=0;
end
end

== matlab function DDCU_wxt_v03/MainControl/mode_control/forward/forward/Drive/驱动防滑控制TCS/转向TCS/右转/前后轮均滑转/HeartBeat1 ==
  data: life_pre input; life output
function life = fcn(life_pre)
%#codegen
life=life_pre+1;
if life>15
    life=0;
end
end

== matlab function DDCU_wxt_v03/MainControl/mode_control/forward/forward/Drive/驱动防滑控制TCS/转向TCS/右转/前轮滑转/HeartBeat1 ==
  data: life_pre input; life output
function life = fcn(life_pre)
%#codegen
life=life_pre+1;
if life>15
    life=0;
end
end

== matlab function DDCU_wxt_v03/MainControl/mode_control/forward/forward/Drive/驱动防滑控制TCS/转向TCS/右转/后轮滑转/HeartBeat1 ==
  data: life_pre input; life output
function life = fcn(life_pre)
%#codegen
life=life_pre+1;
if life>15
    life=0;
end
end

== matlab function DDCU_wxt_v03/MainControl/mode_control/forward/forward/Drive/驱动防滑控制TCS/转向TCS/右转/无滑转/HeartBeat1 ==
  data: life_pre input; life output
function life = fcn(life_pre)
%#codegen
life=life_pre+1;
if life>15
    life=0;
end
end

== matlab function DDCU_wxt_v03/MainControl/mode_control/forward/forward/Drive/驱动防滑控制TCS/转向TCS/左转/MATLAB Function1 ==
  data: s_act_lr input; flag_lr output; s_opt_zhuan input; s_opt_zhuan_add input; flag_lr_pre input
function flag_lr = fcn(s_act_lr,s_opt_zhuan,s_opt_zhuan_add,flag_lr_pre)
%#codegen
if s_act_lr>s_opt_zhuan+s_opt_zhuan_add
    flag_lr=1;
elseif s_act_lr<s_opt_zhuan
    flag_lr = 0;
else
    flag_lr=flag_lr_pre;
end
end

== matlab function DDCU_wxt_v03/MainControl/mode_control/forward/forward/Drive/驱动防滑控制TCS/转向TCS/左转/MATLAB Function3 ==
  data: s_act_rr input; flag_rr output; s_opt_zhuan input; s_opt_zhuan_add input; flag_rr_pre input
function flag_rr = fcn(s_act_rr,s_opt_zhuan,s_opt_zhuan_add,flag_rr_pre)
%#codegen
if s_act_rr>s_opt_zhuan+s_opt_zhuan_add
    flag_rr=1;
elseif s_act_rr<s_opt_zhuan
    flag_rr = 0;
else
    flag_rr=flag_rr_pre;
end
end

== matlab function DDCU_wxt_v03/MainControl/mode_control/forward/forward/Drive/驱动防滑控制TCS/转向TCS/左转/前后轮均滑转/HeartBeat ==
  data: life_pre input; life output
function life = fcn(life_pre)
%#codegen
life=life_pre+1;
if life>15
    life=0;
end
end

== matlab function DDCU_wxt_v03/MainControl/mode_control/forward/forward/Drive/驱动防滑控制TCS/转向TCS/左转/前后轮均滑转/HeartBeat1 ==
  data: life_pre input; life output
function life = fcn(life_pre)
%#codegen
life=life_pre+1;
if life>15
    life=0;
end
end

== matlab function DDCU_wxt_v03/MainControl/mode_control/forward/forward/Drive/驱动防滑控制TCS/转向TCS/左转/前轮滑转/HeartBeat1 ==
  data: life_pre input; life output
function life = fcn(life_pre)
%#codegen
life=life_pre+1;
if life>15
    life=0;
end
end

== matlab function DDCU_wxt_v03/MainControl/mode_control/forward/forward/Drive/驱动防滑控制TCS/转向TCS/左转/后轮滑转/HeartBeat1 ==
  data: life_pre input; life output
function life = fcn(life_pre)
%#codegen
life=life_pre+1;
if life>15
    life=0;
end
end

== matlab function DDCU_wxt_v03/MainControl/mode_control/forward/forward/Drive/驱动防滑控制TCS/转向TCS/左转/无滑转/HeartBeat1 ==
  data: life_pre input; life output
function life = fcn(life_pre)
%#codegen
life=life_pre+1;
if life>15
    life=0;
end
end

== matlab function DDCU_wxt_v03/MainControl/mode_control/neutral/neutral/HeartBeat ==
  data: life_pre input; life output
function life = fcn(life_pre)
%#codegen
life=life_pre+1;
if life>15
    life=0;
end
end

== matlab function DDCU_wxt_v03/MainControl/mode_switch/mode_switch ==
  data: mode_dem input; mode_dem_out output; brake_emerg input; speed_act_lf input; speed_act_lr input; speed_act_rf input; speed_act_rr input; v_act input; v_thr_park input; speed_thr_park input; mode_dem_out_pre input
function mode_dem_out = fcn(mode_dem,brake_emerg,speed_act_lf,speed_act_lr,speed_act_rf,speed_act_rr,v_act,v_thr_park,speed_thr_park,mode_dem_out_pre)
%#codegen
mode_dem_out=mode_dem_out_pre;

if mode_dem==0 && abs(v_act)<=v_thr_park && speed_act_lf<=speed_thr_park && speed_act_lr<=speed_thr_park && speed_act_rf<=speed_thr_park && speed_act_rr<=speed_thr_park && brake_emerg==0
    mode_dem_out=0;
elseif mode_dem==1 && v_act>=-v_thr_park && speed_act_lf>=0 && speed_act_lr>=0 && speed_act_rf>=0 && speed_act_rr>=0 && brake_emerg==0
    mode_dem_out=1;
elseif mode_dem==2 && brake_emerg==0
    mode_dem_out=2;
elseif mode_dem==3 && v_act<=v_thr_park && speed_act_lf>=0 && speed_act_lr>=0 && speed_act_rf>=0 && speed_act_rr>=0 && brake_emerg==0
    mode_dem_out=3;
elseif mode_dem==4 && v_act<=v_thr_park &&  v_act>=-v_thr_park % && speed_act_lf==0 && speed_act_lr==0 && speed_act_rf==0 && speed_act_rr==0 && brake_emerg==0       
    mode_dem_out=4;
elseif brake_emerg==1
    mode_dem_out=5;
% else
%     mode_dem_out=5;
end
end

== system DDCU_wxt_v03/MainControl/mode_control/forward/forward/Drive/驱动防滑控制TCS/转向TCS/右转 ==
  trq_dem_lf : Inport
  trq_dem_lr : Inport  Port=2
  trq_dem_rf : Inport  Port=3
  trq_dem_rr : Inport  Port=4
  bra_pre_l : Inport  Port=5
  bra_pre_r : Inport  Port=6
  s_act_lf : Inport  Port=7
  s_act_lr : Inport  Port=8
  s_act_rf : Inport  Port=9
  s_act_rr : Inport  Port=10
  brake_dem : Inport  Port=11
  s_opt_zhuan : Inport  Port=12
  Action Port : ActionPort
  Constant{,1..3} (4 alike) : Constant  Value=s_opt_zhuan_add
  MATLAB Function : MATLAB Function  TreatAsAtomicUnit=on
  MATLAB Function1 : MATLAB Function  TreatAsAtomicUnit=on
  MATLAB Function2 : MATLAB Function  TreatAsAtomicUnit=on
  MATLAB Function3 : MATLAB Function  TreatAsAtomicUnit=on
  MATLAB Function4 : MATLAB Function  TreatAsAtomicUnit=on
  Memory{,1..3} (4 alike) : Memory  InheritSampleTime=on
  Multiport Switch : MultiPortSwitch  DataPortOrder=Zero-based contiguous  Inputs=4
  Mux{,1..3} (4 alike) : Mux  Inputs=6
  Switch Case : SwitchCase  CaseConditions={0,1,2,3}  ShowDefaultCase=off
  Terminator : Terminator
  Terminator1 : Terminator
  前后轮均滑转 : Subsystem  TreatAsAtomicUnit=on
  前轮滑转 : Subsystem  TreatAsAtomicUnit=on
  后轮滑转 : Subsystem  TreatAsAtomicUnit=on
  无滑转 : Subsystem  TreatAsAtomicUnit=on
  forward_dem : Outport
  wires:
  Mux3/1 -> Multiport Switch/5
  [s_opt_zhuan] -> 前后轮均滑转/10(s_opt_zhuan)
  [s_act_lr] -> 前后轮均滑转/9(s_act_lr)
  [s_act_lf] -> 前后轮均滑转/8(s_act_lf)
  Switch Case/4 -> 前后轮均滑转/Action
  前后轮均滑转/6(bra_pre_r1) -> Mux3/6
  前后轮均滑转/5(bra_pre_l1) -> Mux3/5
  前后轮均滑转/4(mot_rr) -> Mux3/4
  前后轮均滑转/2(mot_lr) -> Mux3/2
  前后轮均滑转/3(mot_rf) -> Mux3/3
  前后轮均滑转/1(mot_lf) -> Mux3/1
  Switch Case/3 -> 后轮滑转/Action
  [s_opt_zhuan] -> 后轮滑转/9(s_opt_zhuan)
  [s_act_lr] -> 后轮滑转/8(s_act_lr)
  Mux2/1 -> Multiport Switch/4
  后轮滑转/6(bra_pre_r1) -> Mux2/6
  后轮滑转/5(bra_pre_l1) -> Mux2/5
  后轮滑转/4(mot_rr) -> Mux2/4
  后轮滑转/2(mot_lr) -> Mux2/2
  后轮滑转/3(mot_rf) -> Mux2/3
  后轮滑转/1(mot_lf) -> Mux2/1
  [s_opt_zhuan] -> 前轮滑转/9(s_opt_zhuan)
  [s_act_lf] -> 前轮滑转/8(s_act_lf)
  Mux1/1 -> Multiport Switch/3
  前轮滑转/4(mot_rr) -> Mux1/4
  前轮滑转/5(bra_pre_l1) -> Mux1/5
  前轮滑转/1(mot_lf) -> Mux1/1
  前轮滑转/2(mot_lr) -> Mux1/2
  前轮滑转/3(mot_rf) -> Mux1/3
  前轮滑转/6(bra_pre_r1) -> Mux1/6
  Switch Case/2 -> 前轮滑转/Action
  Multiport Switch/1 -> forward_dem/1
  Mux/1 -> Multiport Switch/2
  无滑转/6(bra_pre_r1) -> Mux/6
  无滑转/5(bra_pre_l1) -> Mux/5
  无滑转/3(mot_rf) -> Mux/3
  无滑转/4(mot_rr) -> Mux/4
  无滑转/2(mot_lr) -> Mux/2
  无滑转/1(mot_lf) -> Mux/1
  brake_dem/1 -> 前轮滑转/7(brake_dem), 后轮滑转/7(brake_dem), 前后轮均滑转/7(brake_dem), 无滑转/7(brake_dem)
  bra_pre_r/1 -> 前轮滑转/6(bra_pre_r), 后轮滑转/6(bra_pre_r), 前后轮均滑转/6(bra_pre_r), 无滑转/6(bra_pre_r)
  bra_pre_l/1 -> 前轮滑转/5(bra_pre_l), 后轮滑转/5(bra_pre_l), 前后轮均滑转/5(bra_pre_l), 无滑转/5(bra_pre_l)
  trq_dem_rr/1 -> 前轮滑转/4(trq_dem_rr), 后轮滑转/4(trq_dem_rr), 前后轮均滑转/4(trq_dem_rr), 无滑转/4(trq_dem_rr)
  trq_dem_rf/1 -> 前轮滑转/3(trq_dem_rf), 后轮滑转/3(trq_dem_rf), 前后轮均滑转/3(trq_dem_rf), 无滑转/3(trq_dem_rf)
  trq_dem_lr/1 -> 后轮滑转/2(trq_dem_lr), 前后轮均滑转/2(trq_dem_lr), 前轮滑转/2(trq_dem_lr), 无滑转/2(trq_dem_lr)
  trq_dem_lf/1 -> 前轮滑转/1(trq_dem_lf), 后轮滑转/1(trq_dem_lf), 前后轮均滑转/1(trq_dem_lf), 无滑转/1(trq_dem_lf)
  Switch Case/1 -> 无滑转/Action
  MATLAB Function4/1(y) -> Switch Case/1, Multiport Switch/1
  [flag_lr] -> MATLAB Function4/2(flag_lr)
  [flag_lf] -> MATLAB Function4/1(flag_lf)
  Constant3/1 -> MATLAB Function3/3(s_opt_zhuan_add)
  Memory3/1 -> MATLAB Function3/4(flag_rr_pre)
  MATLAB Function3/1(flag_rr) -> Terminator1/1, Memory3/1
  s_opt_zhuan/1 -> MATLAB Function/2(s_opt_zhuan), MATLAB Function1/2(s_opt_zhuan), MATLAB Function2/2(s_opt_zhuan), MATLAB Function3/2(s_opt_zhuan), [s_opt_zhuan]
  s_act_rr/1 -> MATLAB Function3/1(s_act_rr)
  Constant2/1 -> MATLAB Function2/3(s_opt_zhuan_add)
  Memory2/1 -> MATLAB Function2/4(flag_rf_pre)
  MATLAB Function2/1(flag_rf) -> Terminator/1, Memory2/1
  s_act_rf/1 -> MATLAB Function2/1(s_act_rf)
  Constant1/1 -> MATLAB Function1/3(s_opt_zhuan_add)
  Memory1/1 -> MATLAB Function1/4(flag_lr_pre)
  MATLAB Function1/1(flag_lr) -> Memory1/1, [flag_lr]
  s_act_lr/1 -> [s_act_lr], MATLAB Function1/1(s_act_lr)
  Constant/1 -> MATLAB Function/3(s_opt_zhuan_add)
  Memory/1 -> MATLAB Function/4(flag_lf_pre)
  MATLAB Function/1(flag_lf) -> [flag_lf], Memory/1
  s_act_lf/1 -> [s_act_lf], MATLAB Function/1(s_act_lf)

== system DDCU_wxt_v03/MainControl/mode_control/forward/forward/Drive/驱动防滑控制TCS/转向TCS/左转 ==
  trq_dem_lf : Inport
  trq_dem_lr : Inport  Port=2
  trq_dem_rf : Inport  Port=3
  trq_dem_rr : Inport  Port=4
  bra_pre_l : Inport  Port=5
  bra_pre_r : Inport  Port=6
  s_act_lf : Inport  Port=7
  s_act_lr : Inport  Port=8
  s_act_rf : Inport  Port=9
  s_act_rr : Inport  Port=10
  brake_dem : Inport  Port=11
  s_opt_zhuan : Inport  Port=12
  Action Port : ActionPort
  Constant{,1..3} (4 alike) : Constant  Value=s_opt_zhuan_add
  MATLAB Function : MATLAB Function  TreatAsAtomicUnit=on
  MATLAB Function1 : MATLAB Function  TreatAsAtomicUnit=on
  MATLAB Function2 : MATLAB Function  TreatAsAtomicUnit=on
  MATLAB Function3 : MATLAB Function  TreatAsAtomicUnit=on
  MATLAB Function4 : MATLAB Function  TreatAsAtomicUnit=on
  Memory{,1..3} (4 alike) : Memory  InheritSampleTime=on
  Multiport Switch : MultiPortSwitch  DataPortOrder=Zero-based contiguous  Inputs=4
  Mux{,1..3} (4 alike) : Mux  Inputs=6
  Switch Case : SwitchCase  CaseConditions={0,1,2,3}  ShowDefaultCase=off
  Terminator : Terminator
  Terminator1 : Terminator
  前后轮均滑转 : Subsystem  TreatAsAtomicUnit=on
  前轮滑转 : Subsystem  TreatAsAtomicUnit=on
  后轮滑转 : Subsystem  TreatAsAtomicUnit=on
  无滑转 : Subsystem  TreatAsAtomicUnit=on
  forward_dem : Outport
  wires:
  s_act_lf/1 -> MATLAB Function/1(s_act_lf)
  MATLAB Function/1(flag_lf) -> Terminator/1, Memory/1
  Memory/1 -> MATLAB Function/4(flag_lf_pre)
  Constant/1 -> MATLAB Function/3(s_opt_zhuan_add)
  s_act_lr/1 -> MATLAB Function1/1(s_act_lr)
  MATLAB Function1/1(flag_lr) -> Terminator1/1, Memory1/1
  Memory1/1 -> MATLAB Function1/4(flag_lr_pre)
  Constant1/1 -> MATLAB Function1/3(s_opt_zhuan_add)
  s_act_rf/1 -> [s_act_rf], MATLAB Function2/1(s_act_rf)
  MATLAB Function2/1(flag_rf) -> Memory2/1, [flag_rf]
  Memory2/1 -> MATLAB Function2/4(flag_rf_pre)
  Constant2/1 -> MATLAB Function2/3(s_opt_zhuan_add)
  s_act_rr/1 -> [s_act_rr], MATLAB Function3/1(s_act_rr)
  s_opt_zhuan/1 -> [s_opt_zhuan], MATLAB Function3/2(s_opt_zhuan), MATLAB Function2/2(s_opt_zhuan), MATLAB Function1/2(s_opt_zhuan), MATLAB Function/2(s_opt_zhuan)
  MATLAB Function3/1(flag_rr) -> [flag_rr], Memory3/1
  Memory3/1 -> MATLAB Function3/4(flag_rr_pre)
  Constant3/1 -> MATLAB Function3/3(s_opt_zhuan_add)
  [flag_rf] -> MATLAB Function4/1(flag_rf)
  [flag_rr] -> MATLAB Function4/2(flag_rr)
  MATLAB Function4/1(y) -> Multiport Switch/1, Switch Case/1
  Switch Case/1 -> 无滑转/Action
  trq_dem_lf/1 -> 无滑转/1(trq_dem_lf), 前后轮均滑转/1(trq_dem_lf), 后轮滑转/1(trq_dem_lf), 前轮滑转/1(trq_dem_lf)
  trq_dem_lr/1 -> 无滑转/2(trq_dem_lr), 前轮滑转/2(trq_dem_lr), 前后轮均滑转/2(trq_dem_lr), 后轮滑转/2(trq_dem_lr)
  trq_dem_rf/1 -> 无滑转/3(trq_dem_rf), 前后轮均滑转/3(trq_dem_rf), 后轮滑转/3(trq_dem_rf), 前轮滑转/3(trq_dem_rf)
  trq_dem_rr/1 -> 无滑转/4(trq_dem_rr), 前后轮均滑转/4(trq_dem_rr), 后轮滑转/4(trq_dem_rr), 前轮滑转/4(trq_dem_rr)
  bra_pre_l/1 -> 无滑转/5(bra_pre_l), 前后轮均滑转/5(bra_pre_l), 后轮滑转/5(bra_pre_l), 前轮滑转/5(bra_pre_l)
  bra_pre_r/1 -> 无滑转/6(bra_pre_r), 前后轮均滑转/6(bra_pre_r), 后轮滑转/6(bra_pre_r), 前轮滑转/6(bra_pre_r)
  brake_dem/1 -> 无滑转/7(brake_dem), 前后轮均滑转/7(brake_dem), 后轮滑转/7(brake_dem), 前轮滑转/7(brake_dem)
  无滑转/1(mot_lf) -> Mux/1
  无滑转/2(mot_lr) -> Mux/2
  无滑转/4(mot_rr) -> Mux/4
  无滑转/3(mot_rf) -> Mux/3
  无滑转/5(bra_pre_l1) -> Mux/5
  无滑转/6(bra_pre_r1) -> Mux/6
  Mux/1 -> Multiport Switch/2
  Multiport Switch/1 -> forward_dem/1
  Switch Case/2 -> 前轮滑转/Action
  前轮滑转/6(bra_pre_r1) -> Mux1/6
  前轮滑转/3(mot_rf) -> Mux1/3
  前轮滑转/2(mot_lr) -> Mux1/2
  前轮滑转/1(mot_lf) -> Mux1/1
  前轮滑转/5(bra_pre_l1) -> Mux1/5
  前轮滑转/4(mot_rr) -> Mux1/4
  Mux1/1 -> Multiport Switch/3
  [s_act_rf] -> 前轮滑转/8(s_act_rf)
  [s_opt_zhuan] -> 前轮滑转/9(s_opt_zhuan)
  后轮滑转/1(mot_lf) -> Mux2/1
  后轮滑转/3(mot_rf) -> Mux2/3
  后轮滑转/2(mot_lr) -> Mux2/2
  后轮滑转/4(mot_rr) -> Mux2/4
  后轮滑转/5(bra_pre_l1) -> Mux2/5
  后轮滑转/6(bra_pre_r1) -> Mux2/6
  Mux2/1 -> Multiport Switch/4
  [s_act_rr] -> 后轮滑转/8(s_act_rr)
  [s_opt_zhuan] -> 后轮滑转/9(s_opt_zhuan)
  Switch Case/3 -> 后轮滑转/Action
  前后轮均滑转/1(mot_lf) -> Mux3/1
  前后轮均滑转/3(mot_rf) -> Mux3/3
  前后轮均滑转/2(mot_lr) -> Mux3/2
  前后轮均滑转/4(mot_rr) -> Mux3/4
  前后轮均滑转/5(bra_pre_l1) -> Mux3/5
  前后轮均滑转/6(bra_pre_r1) -> Mux3/6
  Switch Case/4 -> 前后轮均滑转/Action
  [s_act_rf] -> 前后轮均滑转/8(s_act_rf)
  [s_act_rr] -> 前后轮均滑转/9(s_act_rr)
  [s_opt_zhuan] -> 前后轮均滑转/10(s_opt_zhuan)
  Mux3/1 -> Multiport Switch/5

== system DDCU_wxt_v03/MainControl/mode_control/backward/backward/Drive/驱动防滑控制TCS/直行TCS/直行/Subsystem ==
  s_opt_zhuan : Inport
  s_act_lf : Inport  Port=2
  s_act_lr : Inport  Port=3
  s_act_rf : Inport  Port=4
  s_act_rr : Inport  Port=5
  flag_lf : Inport  Port=6
  flag_lr : Inport  Port=7
  flag_rf : Inport  Port=8
  flag_rr : Inport  Port=9
  trq_dem_lf : Inport  Port=10
  trq_dem_lr : Inport  Port=11
  trq_dem_rf : Inport  Port=12
  trq_dem_rr : Inport  Port=13
  Add{1..2,5,7} (4 alike) : Sum  Inputs=+++
  Add{3..4,6,8} (4 alike) : Sum
  Difference{,1..3} (4 alike) : simulink/Discrete/Difference  ICPrevInput=0.0  InputProcessing=Inherited  OutMin=[]  OutMax=[]  OutDataType=fixdt(1, 16)  OutScaling=2^-10  DoSatur=off
  Discrete-Time Integrator{,1..3} (4 alike) : DiscreteIntegrator  SampleTime=-1  ICPrevOutput=DiscIntNeverNeededParam  ICPrevScaledInput=DiscIntNeverNeededParam
  Gain{1,4,7,10} (4 alike) : Gain  Gain=kp2
  Gain{2,5,8,11} (4 alike) : Gain  Gain=ki2
  Gain{3,6,9,12} (4 alike) : Gain  Gain=kd2
  Gain{13..16} (4 alike) : Gain  Gain=1/tras_ratio
  Sum{,1..3} (4 alike) : Sum  Inputs=|+-
  Switch{,1..3} (4 alike) : Switch  Criteria=u2 > Threshold  Threshold=0.5
  trq_pid_lf : Outport
  trq_pid_lr : Outport  Port=2
  trq_pid_rf : Outport  Port=3
  trq_pid_rr : Outport  Port=4
  wires:
  Difference2/1 -> Add5/3
  Discrete-Time Integrator2/1 -> Add5/2
  Difference3/1 -> Add7/3
  Discrete-Time Integrator3/1 -> Add7/2
  Difference1/1 -> Add1/3
  Discrete-Time Integrator1/1 -> Add1/2
  Difference/1 -> Add2/3
  Discrete-Time Integrator/1 -> Add2/2
  Add5/1 -> Gain16/1
  Sum2/1 -> Gain7/1, Gain9/1, Gain8/1
  Sum3/1 -> Gain10/1, Gain12/1, Gain11/1
  Add7/1 -> Gain15/1
  Gain6/1 -> Difference1/1
  Add1/1 -> Gain14/1
  Sum1/1 -> Gain4/1, Gain6/1, Gain5/1
  Sum/1 -> Gain1/1, Gain3/1, Gain2/1
  Add2/1 -> Gain13/1
  Switch3/1 -> trq_pid_rf/1
  flag_rf/1 -> Switch3/2
  [s_opt_zhuan] -> Sum3/1
  Gain10/1 -> Add7/1
  Gain11/1 -> Discrete-Time Integrator3/1
  Gain12/1 -> Difference3/1
  s_act_rf/1 -> Sum3/2
  trq_dem_rf/1 -> Add8/2, Switch3/3
  Add8/1 -> Switch3/1
  Switch2/1 -> trq_pid_rr/1
  flag_rr/1 -> Switch2/2
  [s_opt_zhuan] -> Sum2/1
  Gain7/1 -> Add5/1
  Gain8/1 -> Discrete-Time Integrator2/1
  Gain9/1 -> Difference2/1
  s_act_rr/1 -> Sum2/2
  trq_dem_rr/1 -> Add6/2, Switch2/3
  Add6/1 -> Switch2/1
  Switch1/1 -> trq_pid_lr/1
  flag_lr/1 -> Switch1/2
  [s_opt_zhuan] -> Sum1/1
  Gain4/1 -> Add1/1
  Gain5/1 -> Discrete-Time Integrator1/1
  s_act_lr/1 -> Sum1/2
  trq_dem_lr/1 -> Add4/2, Switch1/3
  Add4/1 -> Switch1/1
  Switch/1 -> trq_pid_lf/1
  flag_lf/1 -> Switch/2
  s_opt_zhuan/1 -> Sum/1, [s_opt_zhuan]
  Gain1/1 -> Add2/1
  Gain2/1 -> Discrete-Time Integrator/1
  Gain3/1 -> Difference/1
  s_act_lf/1 -> Sum/2
  trq_dem_lf/1 -> Add3/2, Switch/3
  Add3/1 -> Switch/1
  Gain13/1 -> Add3/1
  Gain14/1 -> Add4/1
  Gain15/1 -> Add8/1
  Gain16/1 -> Add6/1
